simulink model "qint_dh_lqr2"  (Simulink 7.5)
settings: Solver=ode8  StartTime=0.0  StopTime=2000  FixedStep=.002  MaxStep=.02  RelTol=1e-3
InitFcn:
  | Ts=0.02;
undefined symbols (not defined in the file): passive_control, SectorSearch
settings Model: Creator=jporter  LastModifiedBy=jporter
settings OptimizationCC: InitFltsAndDblsToZero=on
settings DebuggingCC: StrictBusMsg=Warning

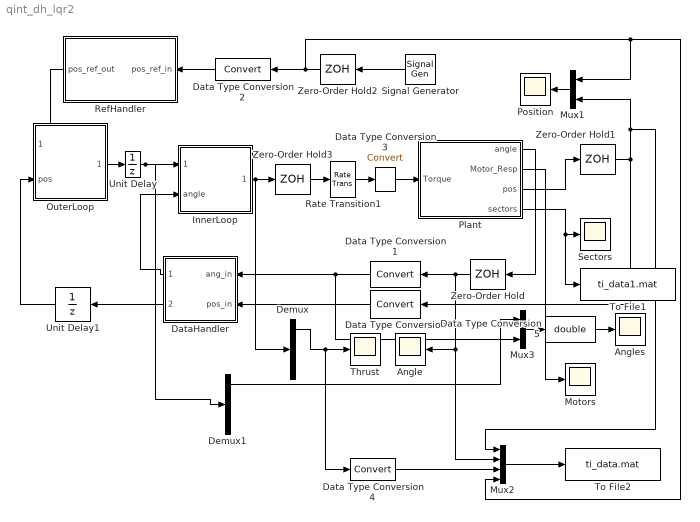
== system qint_dh_lqr2 ==
  Angle : Scope
      settings: YMin=-20  YMax=20
  Angles : Scope
      settings: YMin=-0.2  YMax=0.2  SaveName=ScopeData2
  Data Type Conversion{,1..4} (5 alike) : DataTypeConversion  OutDataType=sfix(16)  OutScaling=2^0
  Data Type Conversion5 : DataTypeConversion  OutDataTypeMode=double  OutDataType=sfix(16)  OutScaling=2^0  OutDataTypeStr=double
  DataHandler : Subsystem
  Demux : Demux  Outputs=9
  Demux1 : Demux  Outputs=5
  InnerLoop : Subsystem
  Motors : Scope
      settings: YMin=-20  YMax=20  SaveName=ScopeData3
  Mux1 : Mux  Inputs=2
  Mux2 : Mux
  Mux3 : Mux  Inputs=2
  OuterLoop : Subsystem
  Plant : Subsystem
  Position : Scope
      settings: YMin=-20  YMax=20
  Rate Transition1 : RateTransition  Priority=0  Integrity=off
  RefHandler : Subsystem
  Sectors : Scope
      settings: YMin=-2  YMax=0  SaveName=ScopeData4
  Signal Generator : SignalGenerator  WaveForm=square  Amplitude=0.5  Frequency=1/30
  Thrust : Scope
      settings: YMin=-20  YMax=20  SaveName=ti_data  DataFormat=Array
  To File1 : ToFile  Filename=ti_data1.mat  MatrixName=sect_data
  To File2 : ToFile  Filename=ti_data.mat  MatrixName=ti_data
  Unit Delay : UnitDelay  SampleTime=-1
  Unit Delay1 : UnitDelay  SampleTime=-1
  Zero-Order Hold : ZeroOrderHold  SampleTime=Ts
  Zero-Order Hold1 : ZeroOrderHold  SampleTime=Ts
  Zero-Order Hold2 : ZeroOrderHold  SampleTime=Ts
  Zero-Order Hold3 : ZeroOrderHold  Priority=-1  SampleTime=-1
  wires:
  InnerLoop/1(Torque) -> Demux/1, Zero-Order Hold3/1
  Plant/3(pos) -> Zero-Order Hold1/1
  Mux1/1 -> Position/1
  Signal Generator/1 -> Zero-Order Hold2/1
  Plant/1(angle) -> Zero-Order Hold/1
  OuterLoop/1(ang_ref) -> Unit Delay/1
  RefHandler/1(pos_ref_out) -> OuterLoop/1(pos_ref)
  Data Type Conversion3/1 -> Plant/1(Torque)
  Zero-Order Hold2/1 -> Data Type Conversion2/1, Mux1/1, Mux2/4
  Zero-Order Hold1/1 -> Data Type Conversion/1, Mux1/2, Mux2/1
  Zero-Order Hold/1 -> Angle/1, Mux2/2, Data Type Conversion1/1
  Data Type Conversion1/1 -> DataHandler/1(ang_in), Mux3/2
  Data Type Conversion/1 -> DataHandler/2(pos_in)
  DataHandler/1(ang_out) -> InnerLoop/2(angle)
  DataHandler/2(pos_out) -> Unit Delay1/1
  Data Type Conversion2/1 -> RefHandler/1(pos_ref_in)
  Plant/2(Motor_Resp) -> Motors/1
  Plant/4(sectors) -> Sectors/1, To File1/1
  Demux/1 -> Thrust/1, Data Type Conversion4/1
  Mux2/1 -> To File2/1
  Data Type Conversion4/1 -> Mux2/3
  Zero-Order Hold3/1 -> Rate Transition1/1
  Rate Transition1/1 -> Data Type Conversion3/1
  Mux3/1 -> Data Type Conversion5/1
  Data Type Conversion5/1 -> Angles/1
  Demux1/1 -> Mux3/1
  Unit Delay/1 -> InnerLoop/1(ang_ref), Demux1/1
  Unit Delay1/1 -> OuterLoop/2(pos)

== system qint_dh_lqr2/DataHandler ==
  ang_in : Inport  PortDimensions=1  DataType=single  OutDataTypeStr=single
  pos_in : Inport  Port=2  PortDimensions=1  DataType=single  OutDataTypeStr=single
  Demux : Demux  Outputs=2
  Mux2 : Mux  Inputs=2
  ang_out : Outport
  pos_out : Outport  Port=2
  wires:
  Mux2/1 -> Demux/1
  Demux/1 -> ang_out/1
  ang_in/1 -> Mux2/1
  Demux/2 -> pos_out/1
  pos_in/1 -> Mux2/2

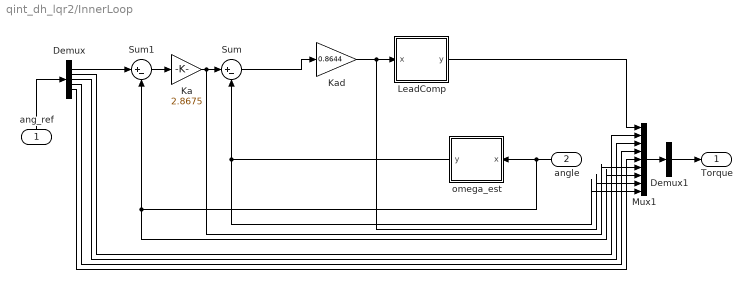
== system qint_dh_lqr2/InnerLoop ==
  ang_ref : Inport  PortDimensions=5  DataType=single  OutDataTypeStr=single
  angle : Inport  Port=2  PortDimensions=1  DataType=single  OutDataTypeStr=single
  Demux : Demux  Outputs=5
  Demux1 : Demux  Outputs=1
  Ka : Gain  Gain=2.8675  ParameterDataTypeMode=single  ParameterDataType=sfix(16)  ParameterScaling=2^0  ParamDataTypeStr=single  OutDataType=sfix(16)  OutScaling=2^0
  Kad : Gain  Gain=0.8644  ParameterDataTypeMode=single  ParameterDataType=sfix(16)  ParameterScaling=2^0  ParamDataTypeStr=single  OutDataType=sfix(16)  OutScaling=2^0
  LeadComp : Subsystem
  Mux1 : Mux  Inputs=9
  Sum : Sum  Inputs=|+-  OutDataType=sfix(16)  OutScaling=2^0
  Sum1 : Sum  Inputs=|+-  OutDataType=sfix(16)  OutScaling=2^0
  omega_est : Subsystem
  Torque : Outport  DataType=single  OutDataTypeStr=single
  wires:
  Sum1/1 -> Ka/1
  Ka/1 -> Sum/1, Mux1/6
  Sum/1 -> Kad/1
  Kad/1 -> LeadComp/1(x), Mux1/8
  omega_est/1(y) -> Sum/2, Mux1/9
  angle/1 -> omega_est/1(x), Sum1/2, Mux1/7
  ang_ref/1 -> Demux/1
  Mux1/1 -> Demux1/1
  Demux/1 -> Sum1/1
  LeadComp/1(y) -> Mux1/1
  Demux/2 -> Mux1/2
  Demux/3 -> Mux1/3
  Demux/4 -> Mux1/4
  Demux/5 -> Mux1/5
  Demux1/1 -> Torque/1

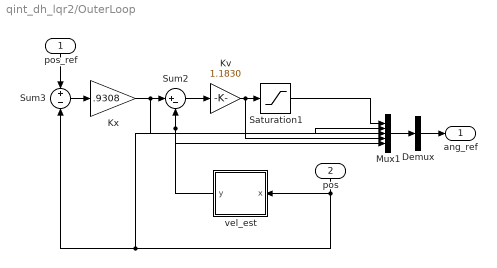
== system qint_dh_lqr2/OuterLoop ==
  pos_ref : Inport  PortDimensions=1  DataType=single  OutDataTypeStr=single
  pos : Inport  Port=2  PortDimensions=1  DataType=single  OutDataTypeStr=single
  Demux : Demux  Outputs=1
  Kv : Gain  Gain=1.1830  ParameterDataTypeMode=single  ParameterDataType=sfix(16)  ParameterScaling=2^0  ParamDataTypeStr=single  OutDataType=sfix(16)  OutScaling=2^0
  Kx : Gain  Gain=.9308  ParameterDataTypeMode=single  ParameterDataType=sfix(16)  ParameterScaling=2^0  ParamDataTypeStr=single  OutDataType=sfix(16)  OutScaling=2^0
  Mux1 : Mux  Inputs=5
  Saturation1 : Saturate  UpperLimit=pi/4  LowerLimit=-pi/4  OutDataType=sfix(16)  OutScaling=2^0
  Sum2 : Sum  Inputs=|+-  OutDataType=sfix(16)  OutScaling=2^0
  Sum3 : Sum  Inputs=+|-  OutDataType=sfix(16)  OutScaling=2^0
  vel_est : Subsystem
  ang_ref : Outport  DataType=single  OutDataTypeStr=single
  wires:
  Kx/1 -> Sum2/1, Mux1/2
  Sum2/1 -> Kv/1
  Kv/1 -> Saturation1/1, Mux1/4
  vel_est/1(y) -> Sum2/2, Mux1/5
  Sum3/1 -> Kx/1
  pos_ref/1 -> Sum3/1
  pos/1 -> vel_est/1(x), Sum3/2, Mux1/3
  Mux1/1 -> Demux/1
  Saturation1/1 -> Mux1/1
  Demux/1 -> ang_ref/1

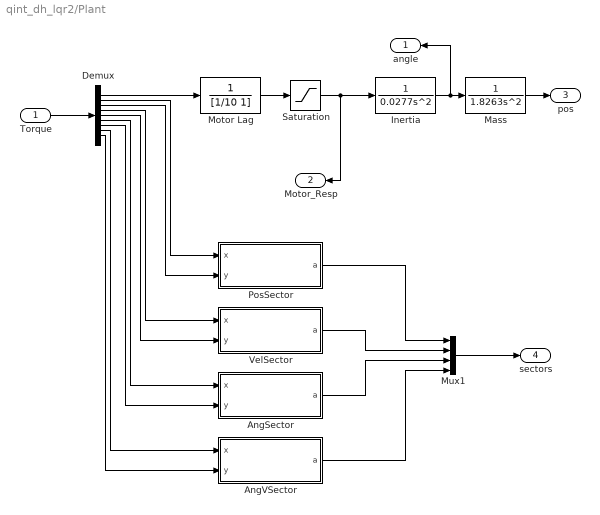
== system qint_dh_lqr2/Plant ==
  Torque : Inport
  AngSector : Subsystem  AncestorBlock=passive_control/SectorSearch
  AngVSector : Subsystem  AncestorBlock=passive_control/SectorSearch
  Demux : Demux  Outputs=9
  Inertia : TransferFcn  Denominator=[0.0277 0 0]
  Mass : TransferFcn  Denominator=[1.8263 0 0]
  Motor Lag : TransferFcn  Denominator=[1/10 1]
  Mux1 : Mux
  PosSector : Subsystem  AncestorBlock=passive_control/SectorSearch
  Saturation : Saturate  UpperLimit=40  LowerLimit=-40  OutDataType=sfix(16)  OutScaling=2^0
  VelSector : Subsystem  AncestorBlock=passive_control/SectorSearch
  angle : Outport
  Motor_Resp : Outport  Port=2
  pos : Outport  Port=3
  sectors : Outport  Port=4
  wires:
  Motor Lag/1 -> Saturation/1
  Saturation/1 -> Inertia/1, Motor_Resp/1
  Inertia/1 -> Mass/1, angle/1
  Mass/1 -> pos/1
  Torque/1 -> Demux/1
  Demux/1 -> Motor Lag/1
  Demux/2 -> PosSector/1(x)
  Demux/3 -> PosSector/2(y)
  Demux/4 -> VelSector/1(x)
  Demux/5 -> VelSector/2(y)
  Demux/6 -> AngSector/1(x)
  Demux/7 -> AngSector/2(y)
  Demux/8 -> AngVSector/1(x)
  Demux/9 -> AngVSector/2(y)
  PosSector/1(a) -> Mux1/1
  VelSector/1(a) -> Mux1/2
  AngSector/1(a) -> Mux1/3
  AngVSector/1(a) -> Mux1/4
  Mux1/1 -> sectors/1

== system qint_dh_lqr2/RefHandler ==
  pos_ref_in : Inport  PortDimensions=1  DataType=single  OutDataTypeStr=single
  rate_limiter : Subsystem  mask{wn=2*pi, zeta=0.9, Vmax=2, T=0.02, Hzn1=0, Hzd1=0}
      mask prompts: wn "omega_n"; Vmax "Max velocity"; T "Sample time"; Hzn1 "Filter numerator"; Hzd1 "Filter denominator"
      mask init:
      | Hs=tf([wn^2],[1,2*zeta*wn,wn^2]);
      | Hz=ipesh_transform(Hs,T);
      | Hzn1 = Hz.num{1};
      | %Hzn1 = [0.002488 0.009405 0.002222];
      | Hzd1 = Hz.den{1};
      | %Hzd1 = [1.0000 -1.7834 0.7976];
  pos_ref_out : Outport
  wires:
  rate_limiter/1(Xr_set) -> pos_ref_out/1
  pos_ref_in/1 -> rate_limiter/1(Xe_set)

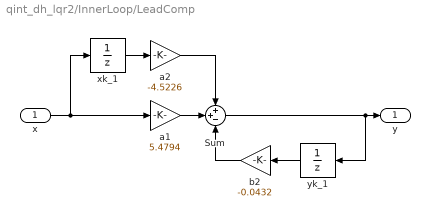
== system qint_dh_lqr2/InnerLoop/LeadComp ==
  x : Inport  PortDimensions=1  DataType=single  OutDataType=sfix(16)  OutScaling=2^0  OutDataTypeStr=single
  Sum : Sum  Inputs=++-  OutDataType=sfix(16)  OutScaling=2^0
  a1 : Gain  Gain=5.4794  ParameterDataTypeMode=single  ParameterDataType=sfix(16)  ParameterScaling=2^0  ParamDataTypeStr=single  OutDataType=sfix(16)  OutScaling=2^0
  a2 : Gain  Gain=-4.5226  ParameterDataTypeMode=single  ParameterDataType=sfix(16)  ParameterScaling=2^0  ParamDataTypeStr=single  OutDataType=sfix(16)  OutScaling=2^0
  b2 : Gain  Gain=-0.0432  ParameterDataTypeMode=single  ParameterDataType=sfix(16)  ParameterScaling=2^0  ParamDataTypeStr=single  OutDataType=sfix(16)  OutScaling=2^0
  xk_1 : UnitDelay  SampleTime=Ts
  yk_1 : UnitDelay  SampleTime=Ts
  y : Outport  OutDataType=sfix(16)  OutScaling=2^0
  wires:
  b2/1 -> Sum/3
  yk_1/1 -> b2/1
  Sum/1 -> y/1, yk_1/1
  a1/1 -> Sum/2
  a2/1 -> Sum/1
  xk_1/1 -> a2/1
  x/1 -> xk_1/1, a1/1

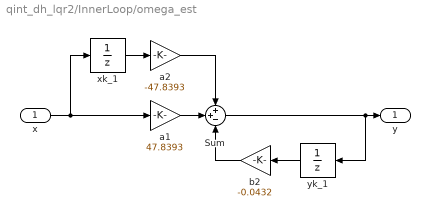
== system qint_dh_lqr2/InnerLoop/omega_est ==
  x : Inport  PortDimensions=1  DataType=single  OutDataType=sfix(16)  OutScaling=2^0  OutDataTypeStr=single
  Sum : Sum  Inputs=++-  OutDataType=sfix(16)  OutScaling=2^0
  a1 : Gain  Gain=47.8393  ParameterDataTypeMode=single  ParameterDataType=sfix(16)  ParameterScaling=2^0  ParamDataTypeStr=single  OutDataType=sfix(16)  OutScaling=2^0
  a2 : Gain  Gain=-47.8393  ParameterDataTypeMode=single  ParameterDataType=sfix(16)  ParameterScaling=2^0  ParamDataTypeStr=single  OutDataType=sfix(16)  OutScaling=2^0
  b2 : Gain  Gain=-0.0432  ParameterDataTypeMode=single  ParameterDataType=sfix(16)  ParameterScaling=2^0  ParamDataTypeStr=single  OutDataType=sfix(16)  OutScaling=2^0
  xk_1 : UnitDelay  SampleTime=Ts
  yk_1 : UnitDelay  SampleTime=Ts
  y : Outport  OutDataType=sfix(16)  OutScaling=2^0
  wires:
  b2/1 -> Sum/3
  yk_1/1 -> b2/1
  Sum/1 -> y/1, yk_1/1
  a1/1 -> Sum/2
  a2/1 -> Sum/1
  xk_1/1 -> a2/1
  x/1 -> xk_1/1, a1/1

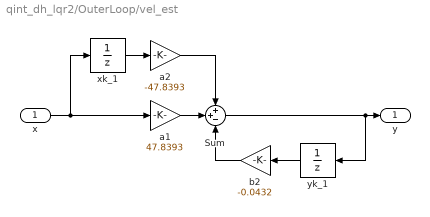
== system qint_dh_lqr2/OuterLoop/vel_est ==
  x : Inport  PortDimensions=1  DataType=single  OutDataType=sfix(16)  OutScaling=2^0  OutDataTypeStr=single
  Sum : Sum  Inputs=++-  OutDataType=sfix(16)  OutScaling=2^0
  a1 : Gain  Gain=47.8393  ParameterDataTypeMode=single  ParameterDataType=sfix(16)  ParameterScaling=2^0  ParamDataTypeStr=single  OutDataType=sfix(16)  OutScaling=2^0
  a2 : Gain  Gain=-47.8393  ParameterDataTypeMode=single  ParameterDataType=sfix(16)  ParameterScaling=2^0  ParamDataTypeStr=single  OutDataType=sfix(16)  OutScaling=2^0
  b2 : Gain  Gain=-0.0432  ParameterDataTypeMode=single  ParameterDataType=sfix(16)  ParameterScaling=2^0  ParamDataTypeStr=single  OutDataType=sfix(16)  OutScaling=2^0
  xk_1 : UnitDelay  SampleTime=Ts
  yk_1 : UnitDelay  SampleTime=Ts
  y : Outport  OutDataType=sfix(16)  OutScaling=2^0
  wires:
  x/1 -> a1/1, xk_1/1
  xk_1/1 -> a2/1
  a2/1 -> Sum/1
  a1/1 -> Sum/2
  Sum/1 -> yk_1/1, y/1
  yk_1/1 -> b2/1
  b2/1 -> Sum/3

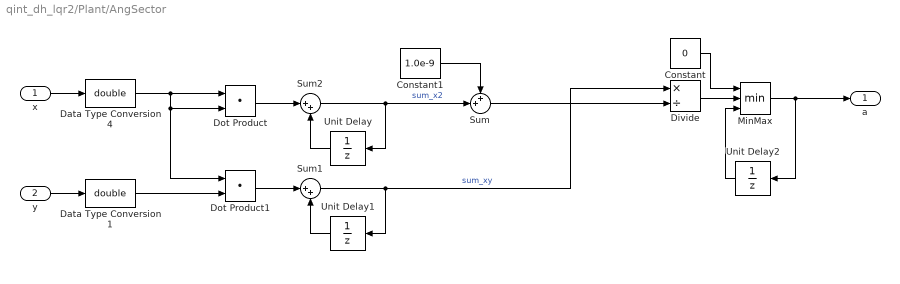
== system qint_dh_lqr2/Plant/AngSector ==
  x : Inport  OutDataType=sfix(16)  OutScaling=2^0
  y : Inport  Port=2  OutDataType=sfix(16)  OutScaling=2^0
  Constant : Constant  Value=0  OutDataTypeMode=double  OutDataType=sfix(16)  OutScaling=2^0  OutDataTypeStr=double
  Constant1 : Constant  Value=1.0e-9  OutDataTypeMode=double  OutDataType=sfix(16)  OutScaling=2^0  OutDataTypeStr=double
  Data Type Conversion1 : DataTypeConversion  OutDataTypeMode=double  OutDataType=sfix(16)  OutScaling=2^0  OutDataTypeStr=double
  Data Type Conversion4 : DataTypeConversion  OutDataTypeMode=double  OutDataType=sfix(16)  OutScaling=2^0  OutDataTypeStr=double
  Divide : Product  Inputs=*/  OutDataType=sfix(16)  OutScaling=2^-10
  Dot Product : DotProduct  OutDataType=sfix(16)  OutScaling=2^-10  InputSameDT=on  OutDataTypeStr=Inherit: Inherit via internal rule
  Dot Product1 : DotProduct  OutDataType=sfix(16)  OutScaling=2^-10  InputSameDT=on  OutDataTypeStr=Inherit: Inherit via internal rule
  MinMax : MinMax  Inputs=3  OutDataTypeMode=double  OutDataType=sfix(16)  OutScaling=2^0  OutDataTypeStr=double
  Sum : Sum  Inputs=++|  OutDataType=sfix(16)  OutScaling=2^0
  Sum1 : Sum  Inputs=|++  OutDataType=sfix(16)  OutScaling=2^0
  Sum2 : Sum  Inputs=|++  OutDataType=sfix(16)  OutScaling=2^0
  Unit Delay : UnitDelay  SampleTime=-1
  Unit Delay1 : UnitDelay  SampleTime=-1
  Unit Delay2 : UnitDelay  SampleTime=-1
  a : Outport  OutDataType=sfix(16)  OutScaling=2^0
  wires:
  Constant1/1 -> Sum/1
  Sum/1 -> Divide/2
  Unit Delay2/1 -> MinMax/3
  Divide/1 -> MinMax/2
  Constant/1 -> MinMax/1
  MinMax/1 -> Unit Delay2/1, a/1
  y/1 -> Data Type Conversion1/1
  x/1 -> Data Type Conversion4/1
  Dot Product1/1 -> Sum1/1
  Unit Delay1/1 -> Sum1/2
  Sum1/1 -> Divide/1, Unit Delay1/1  "sum_xy"
  Dot Product/1 -> Sum2/1
  Unit Delay/1 -> Sum2/2
  Sum2/1 -> Sum/2, Unit Delay/1  "sum_x2"
  Data Type Conversion4/1 -> Dot Product1/1, Dot Product/2, Dot Product/1
  Data Type Conversion1/1 -> Dot Product1/2

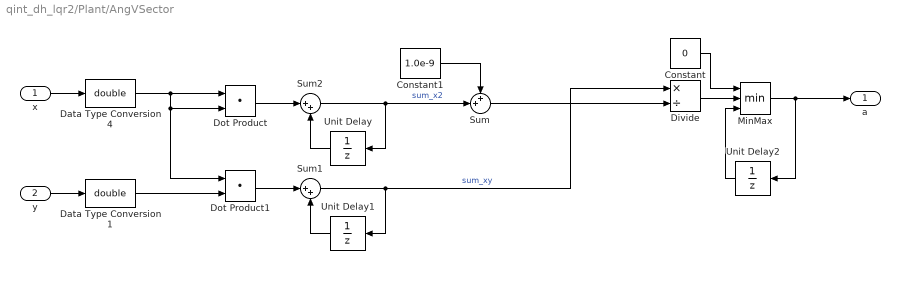
== system qint_dh_lqr2/Plant/AngVSector ==
  x : Inport  OutDataType=sfix(16)  OutScaling=2^0
  y : Inport  Port=2  OutDataType=sfix(16)  OutScaling=2^0
  Constant : Constant  Value=0  OutDataTypeMode=double  OutDataType=sfix(16)  OutScaling=2^0  OutDataTypeStr=double
  Constant1 : Constant  Value=1.0e-9  OutDataTypeMode=double  OutDataType=sfix(16)  OutScaling=2^0  OutDataTypeStr=double
  Data Type Conversion1 : DataTypeConversion  OutDataTypeMode=double  OutDataType=sfix(16)  OutScaling=2^0  OutDataTypeStr=double
  Data Type Conversion4 : DataTypeConversion  OutDataTypeMode=double  OutDataType=sfix(16)  OutScaling=2^0  OutDataTypeStr=double
  Divide : Product  Inputs=*/  OutDataType=sfix(16)  OutScaling=2^-10
  Dot Product : DotProduct  OutDataType=sfix(16)  OutScaling=2^-10  InputSameDT=on  OutDataTypeStr=Inherit: Inherit via internal rule
  Dot Product1 : DotProduct  OutDataType=sfix(16)  OutScaling=2^-10  InputSameDT=on  OutDataTypeStr=Inherit: Inherit via internal rule
  MinMax : MinMax  Inputs=3  OutDataTypeMode=double  OutDataType=sfix(16)  OutScaling=2^0  OutDataTypeStr=double
  Sum : Sum  Inputs=++|  OutDataType=sfix(16)  OutScaling=2^0
  Sum1 : Sum  Inputs=|++  OutDataType=sfix(16)  OutScaling=2^0
  Sum2 : Sum  Inputs=|++  OutDataType=sfix(16)  OutScaling=2^0
  Unit Delay : UnitDelay  SampleTime=-1
  Unit Delay1 : UnitDelay  SampleTime=-1
  Unit Delay2 : UnitDelay  SampleTime=-1
  a : Outport  OutDataType=sfix(16)  OutScaling=2^0
  wires:
  Constant1/1 -> Sum/1
  Sum/1 -> Divide/2
  Unit Delay2/1 -> MinMax/3
  Divide/1 -> MinMax/2
  Constant/1 -> MinMax/1
  MinMax/1 -> Unit Delay2/1, a/1
  y/1 -> Data Type Conversion1/1
  x/1 -> Data Type Conversion4/1
  Dot Product1/1 -> Sum1/1
  Unit Delay1/1 -> Sum1/2
  Sum1/1 -> Divide/1, Unit Delay1/1  "sum_xy"
  Dot Product/1 -> Sum2/1
  Unit Delay/1 -> Sum2/2
  Sum2/1 -> Sum/2, Unit Delay/1  "sum_x2"
  Data Type Conversion4/1 -> Dot Product1/1, Dot Product/2, Dot Product/1
  Data Type Conversion1/1 -> Dot Product1/2

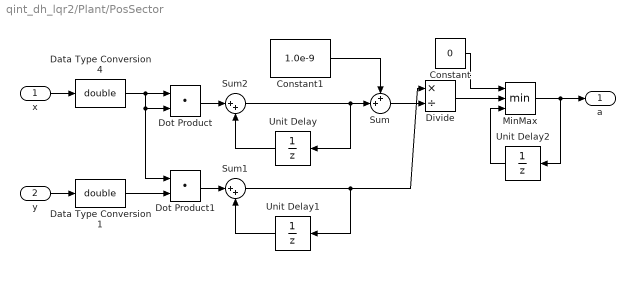
== system qint_dh_lqr2/Plant/PosSector ==
  x : Inport  OutDataType=sfix(16)  OutScaling=2^0
  y : Inport  Port=2  OutDataType=sfix(16)  OutScaling=2^0
  Constant : Constant  Value=0  OutDataTypeMode=double  OutDataType=sfix(16)  OutScaling=2^0  OutDataTypeStr=double
  Constant1 : Constant  Value=1.0e-9  OutDataTypeMode=double  OutDataType=sfix(16)  OutScaling=2^0  OutDataTypeStr=double
  Data Type Conversion1 : DataTypeConversion  OutDataTypeMode=double  OutDataType=sfix(16)  OutScaling=2^0  OutDataTypeStr=double
  Data Type Conversion4 : DataTypeConversion  OutDataTypeMode=double  OutDataType=sfix(16)  OutScaling=2^0  OutDataTypeStr=double
  Divide : Product  Inputs=*/  OutDataType=sfix(16)  OutScaling=2^-10
  Dot Product : DotProduct  OutDataType=sfix(16)  OutScaling=2^-10  InputSameDT=on  OutDataTypeStr=Inherit: Inherit via internal rule
  Dot Product1 : DotProduct  OutDataType=sfix(16)  OutScaling=2^-10  InputSameDT=on  OutDataTypeStr=Inherit: Inherit via internal rule
  MinMax : MinMax  Inputs=3  OutDataTypeMode=double  OutDataType=sfix(16)  OutScaling=2^0  OutDataTypeStr=double
  Sum : Sum  Inputs=++|  OutDataType=sfix(16)  OutScaling=2^0
  Sum1 : Sum  Inputs=|++  OutDataType=sfix(16)  OutScaling=2^0
  Sum2 : Sum  Inputs=|++  OutDataType=sfix(16)  OutScaling=2^0
  Unit Delay : UnitDelay  SampleTime=-1
  Unit Delay1 : UnitDelay  SampleTime=-1
  Unit Delay2 : UnitDelay  SampleTime=-1
  a : Outport  OutDataType=sfix(16)  OutScaling=2^0
  wires:
  Constant1/1 -> Sum/1
  Sum/1 -> Divide/2
  Unit Delay2/1 -> MinMax/3
  Divide/1 -> MinMax/2
  Constant/1 -> MinMax/1
  MinMax/1 -> Unit Delay2/1, a/1
  y/1 -> Data Type Conversion1/1
  x/1 -> Data Type Conversion4/1
  Dot Product1/1 -> Sum1/1
  Unit Delay1/1 -> Sum1/2
  Sum1/1 -> Divide/1, Unit Delay1/1
  Dot Product/1 -> Sum2/1
  Unit Delay/1 -> Sum2/2
  Sum2/1 -> Sum/2, Unit Delay/1
  Data Type Conversion4/1 -> Dot Product1/1, Dot Product/2, Dot Product/1
  Data Type Conversion1/1 -> Dot Product1/2

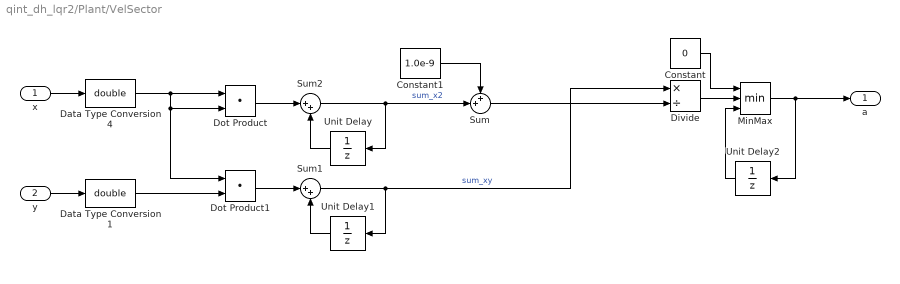
== system qint_dh_lqr2/Plant/VelSector ==
  x : Inport  OutDataType=sfix(16)  OutScaling=2^0
  y : Inport  Port=2  OutDataType=sfix(16)  OutScaling=2^0
  Constant : Constant  Value=0  OutDataTypeMode=double  OutDataType=sfix(16)  OutScaling=2^0  OutDataTypeStr=double
  Constant1 : Constant  Value=1.0e-9  OutDataTypeMode=double  OutDataType=sfix(16)  OutScaling=2^0  OutDataTypeStr=double
  Data Type Conversion1 : DataTypeConversion  OutDataTypeMode=double  OutDataType=sfix(16)  OutScaling=2^0  OutDataTypeStr=double
  Data Type Conversion4 : DataTypeConversion  OutDataTypeMode=double  OutDataType=sfix(16)  OutScaling=2^0  OutDataTypeStr=double
  Divide : Product  Inputs=*/  OutDataType=sfix(16)  OutScaling=2^-10
  Dot Product : DotProduct  OutDataType=sfix(16)  OutScaling=2^-10  InputSameDT=on  OutDataTypeStr=Inherit: Inherit via internal rule
  Dot Product1 : DotProduct  OutDataType=sfix(16)  OutScaling=2^-10  InputSameDT=on  OutDataTypeStr=Inherit: Inherit via internal rule
  MinMax : MinMax  Inputs=3  OutDataTypeMode=double  OutDataType=sfix(16)  OutScaling=2^0  OutDataTypeStr=double
  Sum : Sum  Inputs=++|  OutDataType=sfix(16)  OutScaling=2^0
  Sum1 : Sum  Inputs=|++  OutDataType=sfix(16)  OutScaling=2^0
  Sum2 : Sum  Inputs=|++  OutDataType=sfix(16)  OutScaling=2^0
  Unit Delay : UnitDelay  SampleTime=-1
  Unit Delay1 : UnitDelay  SampleTime=-1
  Unit Delay2 : UnitDelay  SampleTime=-1
  a : Outport  OutDataType=sfix(16)  OutScaling=2^0
  wires:
  Constant1/1 -> Sum/1
  Sum/1 -> Divide/2
  Unit Delay2/1 -> MinMax/3
  Divide/1 -> MinMax/2
  Constant/1 -> MinMax/1
  MinMax/1 -> Unit Delay2/1, a/1
  y/1 -> Data Type Conversion1/1
  x/1 -> Data Type Conversion4/1
  Dot Product1/1 -> Sum1/1
  Unit Delay1/1 -> Sum1/2
  Sum1/1 -> Divide/1, Unit Delay1/1  "sum_xy"
  Dot Product/1 -> Sum2/1
  Unit Delay/1 -> Sum2/2
  Sum2/1 -> Sum/2, Unit Delay/1  "sum_x2"
  Data Type Conversion4/1 -> Dot Product1/1, Dot Product/2, Dot Product/1
  Data Type Conversion1/1 -> Dot Product1/2

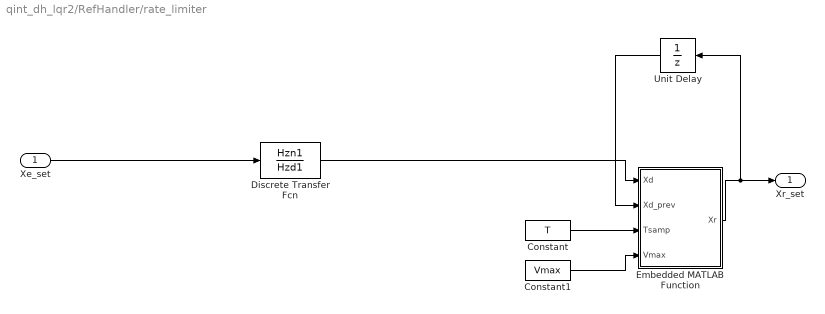
== system qint_dh_lqr2/RefHandler/rate_limiter ==
  Xe_set : Inport  OutDataType=sfix(16)  OutScaling=2^0
  Constant : Constant  Value=T  OutDataTypeMode=single  OutDataType=sfix(16)  OutScaling=2^0  OutDataTypeStr=single
  Constant1 : Constant  Value=Vmax  OutDataTypeMode=single  OutDataType=sfix(16)  OutScaling=2^0  OutDataTypeStr=single
  Discrete Transfer Fcn : DiscreteTransferFcn  Numerator=Hzn1  Denominator=Hzd1  SampleTime=-1
  Embedded MATLAB Function : Stateflow chart  TreatAsAtomicUnit=on
  Unit Delay : UnitDelay  SampleTime=-1
  Xr_set : Outport  OutDataType=sfix(16)  OutScaling=2^0
  wires:
  Embedded MATLAB Function/1(Xr) -> Xr_set/1, Unit Delay/1
  Unit Delay/1 -> Embedded MATLAB Function/2(Xd_prev)
  Constant/1 -> Embedded MATLAB Function/3(Tsamp)
  Constant1/1 -> Embedded MATLAB Function/4(Vmax)
  Xe_set/1 -> Discrete Transfer Fcn/1
  Discrete Transfer Fcn/1 -> Embedded MATLAB Function/1(Xd)

== matlab function RefHandler/rate_limiter/Embedded MATLAB Function ==
  data: Xd input single; Xr output single; Xd_prev input single; Tsamp input single size=[1]; Vmax input single size=[1]
function Xr = limit_rate(Xd, Xd_prev, Tsamp, Vmax)
% This block supports the Embedded MATLAB subset.
% See the help menu for details. 

delta = Xd - Xd_prev;
delta = sign(delta) .* min( abs(delta), (Tsamp * Vmax) );

Xr = Xd_prev + delta;
